simulink model "step_contoller"  (R2023a)
settings: Solver=VariableStepAuto  StartTime=0.0  StopTime=100  RelTol=1e-3
settings Model: Creator=User  LastModifiedBy=User

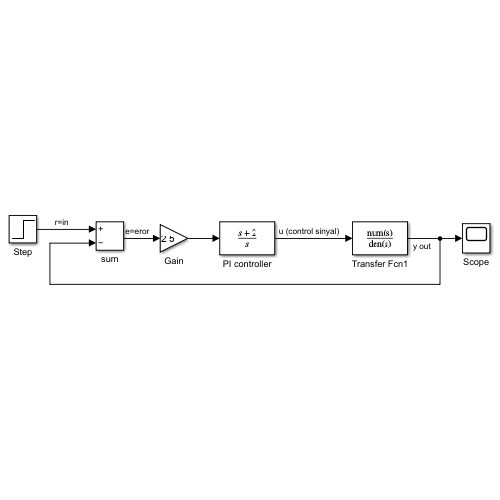
[thumbnail: Simulink's stored preview of the top-level diagram]
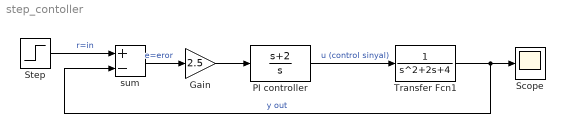
== system step_contoller ==
  Gain : Gain  Gain=2.5
  PI controller : TransferFcn  Numerator=[1 2]  Denominator=[1 0]
  Scope : Scope
  Step : Step  SampleTime=0
  Transfer Fcn1 : TransferFcn  Denominator=[1 2 4]
  sum : Sum  Inputs=+-
  wires:
  PI controller/1 -> Transfer Fcn1/1  "u (control sinyal)"
  Gain/1 -> PI controller/1
  sum/1 -> Gain/1  "e=eror"
  Transfer Fcn1/1 -> Scope/1, sum/2  "y out"
  Step/1 -> sum/1  "r=in"
